simulink model "KukaSimModel"  (R2024b)
settings: Solver=VariableStepAuto  StartTime=0.0  StopTime=30  FixedStep=0.01  RelTol=1e-3
PreLoadFcn:
  | TP_TASK_SPACE = Simulink.Variant('TP_MODE==1');
  | TP_JOINT_SPACE = Simulink.Variant('TP_MODE==2');
InitFcn:
  | printlog('Start simulation...');
  | 
  | if TP_MODE == 1
  |     printlog('Run simulation...');
  |     return;
  | end
  | 
  | printlog('Solve Inverse Kinematics in JointSpace...');
  | jointWaypoints = zeros(6, size(waypointsStruct.waypoints, 2));
  | for i=1:size(waypointsStruct.waypoints, 2)
  |     if isempty(waypointsStruct.orientations)
  |         R = eye(3, 3);
  |     else
  |         R = trajectory.convertEulerToRotationMatrix(waypointsStruct.orientations(:, i));
  |     end
  |     % create homogeneous transform for inverse kinematics
  |     T = [R, waypointsStruct.waypoints(:, i); zeros(1, 3), 1];
  |     jointWaypoints(:, i) = solver.solveInverseKinematics(dhParametersStruct, T);
  | end
  | printlog('Run simulation...');
StopFcn:
  | t = datetime('now');
  | printlog('Stop simulation.');
undefined symbols (not defined in the file): dhParametersStruct, dt_FixedStep, dynamicParametersStruct, q1, q2, q3, q4, q5, q6, tau1, tau2, tau3, tau4, tau5, tau6, waypointsStruct
libraries: lib_Solver x5
settings Model: Creator=chiar  LastModifiedBy=Collins
settings OptimizationCC: BlockReduction=off  DefaultParameterBehavior=Inlined  BufferReuse=off
settings DebuggingCC: UnconnectedInputMsg=warning  UnconnectedOutputMsg=warning  UnconnectedLineMsg=warning
settings ModelReferenceCC: EnableRefExpFcnMdlSchedulingChecks=on
settings RTWCC: GPUComputeCapability=3.5  DLArmComputeVersion=19.05
settings GRTTargetCC: RTWCAPISignals=on  RTWCAPIParams=on

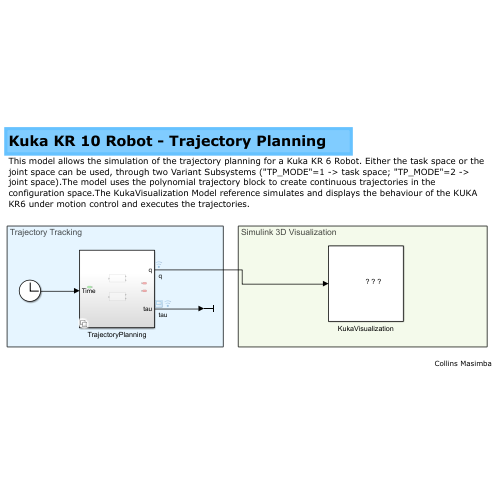
[thumbnail: Simulink's stored preview of the top-level diagram]
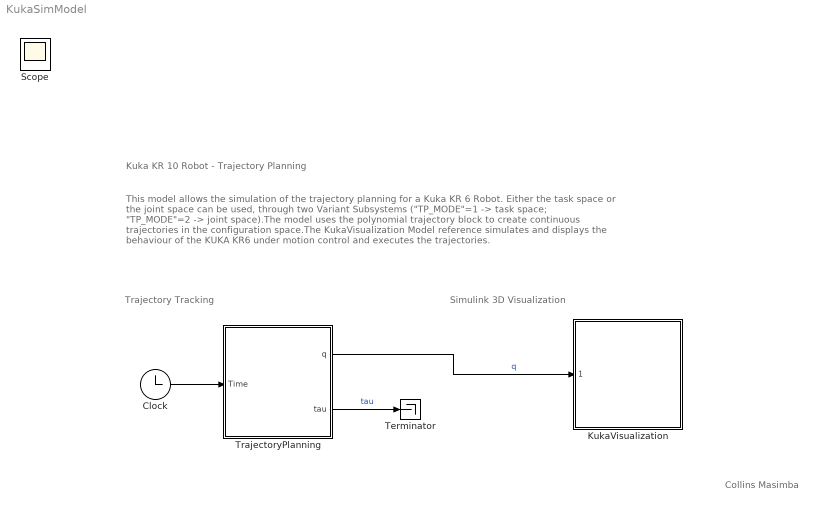
== system KukaSimModel ==
  note: Collins Masimba
  note: Trajectory Tracking
  note: Simulink 3D Visualization
  note: This model allows the simulation of the trajectory planning for a Kuka KR 6 Robot. Either the task space or the joint space can be used, through two Variant Subsystems ("TP_MODE"=1 -> task space; "TP_MODE"=2 -> joint space).The model uses the polynomial trajectory block to create continuous trajectories in the configuration space.The KukaVisualization Model reference simulates and displays the behaviour of the KUKA KR6 under motion control and executes the trajectories.
  note: Kuka KR 10 Robot - Trajectory Planning
  Clock : Clock
  KukaVisualization : Subsystem  ReferencedSubsystem=KukaVisualizationModel
  Terminator : Terminator
  TrajectoryPlanning : Subsystem  Variant=on
  Scope : Scope
  wires:
  TrajectoryPlanning/1(q) -> KukaVisualization/1  "q"
  Clock/1 -> TrajectoryPlanning/1(Time)
  TrajectoryPlanning/2(tau) -> Terminator/1  "tau"

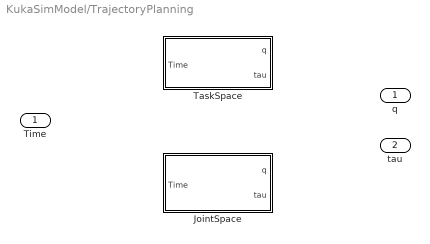
== system KukaSimModel/TrajectoryPlanning ==
  Time : Inport
  JointSpace : Subsystem  VariantControl=TP_MODE == 2
  TaskSpace : Subsystem  VariantControl=TP_MODE == 1
  q : Outport  OutDataTypeStr=Bus: Bus_q
  tau : Outport  Port=2  OutDataTypeStr=double

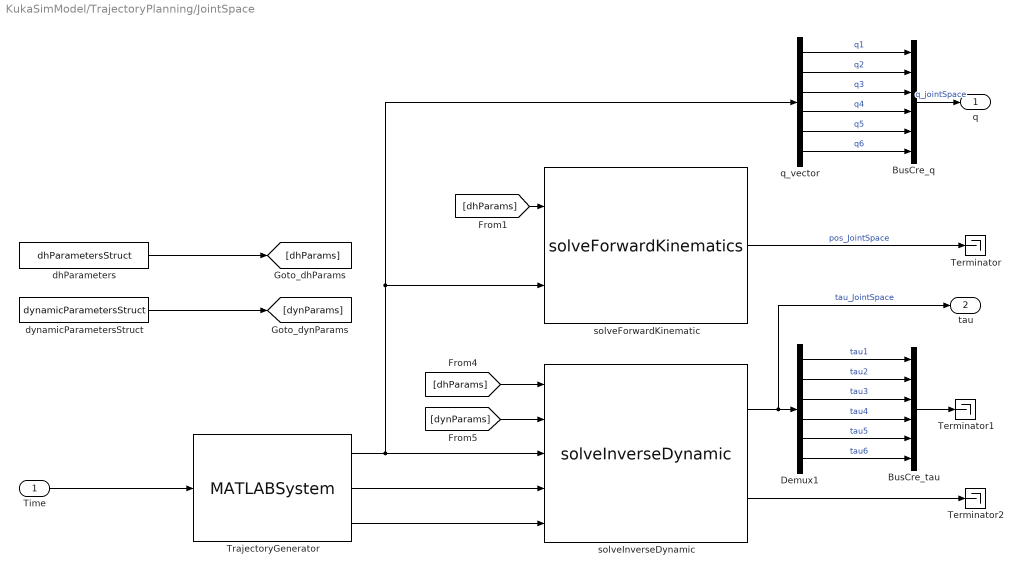
== system KukaSimModel/TrajectoryPlanning/JointSpace ==
  Time : Inport
  BusCre_q : BusCreator  Inputs=q1,q2,q3,q4,q5,q6  OutDataTypeStr=Bus: Bus_q
  BusCre_tau : BusCreator  Inputs=tau1,tau2,tau3,tau4,tau5,tau6  OutDataTypeStr=Bus: Bus_tau
  Demux1 : Demux  Outputs=6
  Terminator : Terminator
  Terminator1 : Terminator
  Terminator2 : Terminator
  TrajectoryGenerator : MATLABSystem  System=core.TrajectoryGenerator  SolverSpace=JointSpace  Method=Cubic Polynomial  Waypoints=jointWaypoints  Timepoints=waypointsStruct.times  Velocities=zeros(6, size(waypointsStruct.waypoints, 2))  Accelerations=zeros(6, size(waypointsStruct.waypoints, 2))  Orientations=zeros( 3, 5 )  PropertyLogical=off  SimulateUsing=Interpreted execution
  dhParameters : Constant  Value=dhParametersStruct  OutDataTypeStr=Bus: Bus_dhParameter
  dynamicParametersStruct : Constant  Value=dynamicParametersStruct  OutDataTypeStr=Bus: Bus_dynamicsParameter
  q_vector : Demux  Outputs=6
  solveForwardKinematic : lib_Solver/solveForwardKinematics  SystemSampleTime=-1  VariantActivationTime=update diagram  Latency=0  AutoFrameSizeCalculation=off
  solveInverseDynamic : lib_Solver/solveInverseDynamic  SystemSampleTime=-1  VariantActivationTime=update diagram  Latency=0  AutoFrameSizeCalculation=off
  q : Outport  OutDataTypeStr=Bus: Bus_q
  tau : Outport  Port=2  OutDataTypeStr=double
  wires:
  Time/1 -> TrajectoryGenerator/1
  [dynParams] -> solveInverseDynamic/2
  [dhParams] -> solveInverseDynamic/1
  solveInverseDynamic/1 -> tau/1, Demux1/1  "tau_JointSpace"
  q_vector/6 -> BusCre_q/6  "q6"
  q_vector/1 -> BusCre_q/1  "q1"
  q_vector/2 -> BusCre_q/2  "q2"
  q_vector/3 -> BusCre_q/3  "q3"
  q_vector/5 -> BusCre_q/5  "q5"
  q_vector/4 -> BusCre_q/4  "q4"
  TrajectoryGenerator/1 -> solveInverseDynamic/3, q_vector/1, solveForwardKinematic/2
  BusCre_q/1 -> q/1  "q_jointSpace"
  solveInverseDynamic/2 -> Terminator2/1
  dhParameters/1 -> [dhParams]
  dynamicParametersStruct/1 -> [dynParams]
  [dhParams] -> solveForwardKinematic/1
  solveForwardKinematic/1 -> Terminator/1  "pos_JointSpace"
  TrajectoryGenerator/2 -> solveInverseDynamic/4
  TrajectoryGenerator/3 -> solveInverseDynamic/5
  Demux1/4 -> BusCre_tau/4  "tau4"
  Demux1/5 -> BusCre_tau/5  "tau5"
  Demux1/3 -> BusCre_tau/3  "tau3"
  Demux1/1 -> BusCre_tau/1  "tau1"
  Demux1/6 -> BusCre_tau/6  "tau6"
  Demux1/2 -> BusCre_tau/2  "tau2"
  BusCre_tau/1 -> Terminator1/1

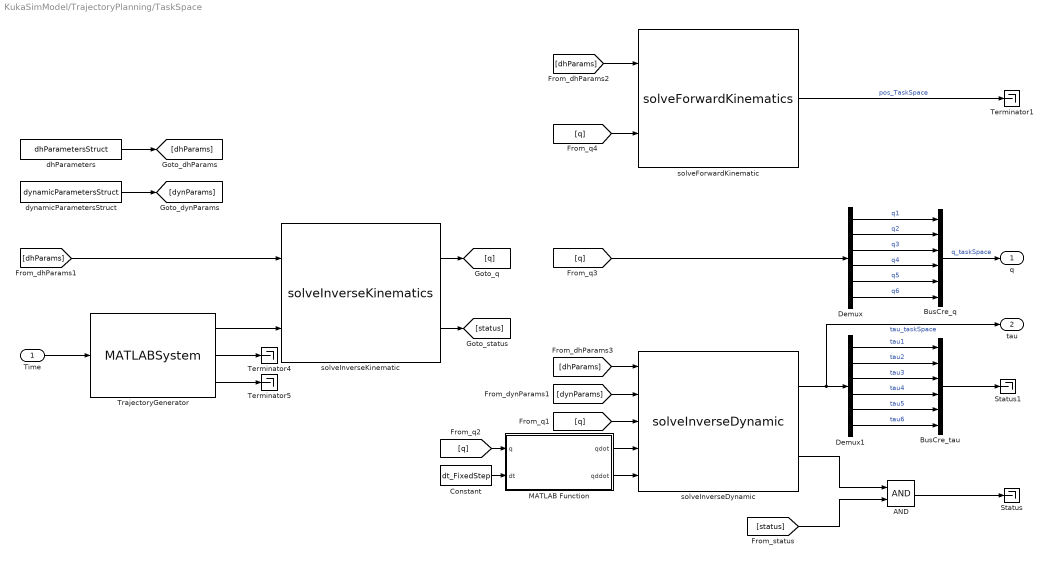
== system KukaSimModel/TrajectoryPlanning/TaskSpace ==
  Time : Inport
  AND : Logic  AllPortsSameDT=off  OutDataTypeStr=boolean
  BusCre_q : BusCreator  Inputs=q1,q2,q3,q4,q5,q6  OutDataTypeStr=Bus: Bus_q
  BusCre_tau : BusCreator  Inputs=tau1,tau2,tau3,tau4,tau5,tau6  OutDataTypeStr=Bus: Bus_tau
  Constant : Constant  Value=dt_FixedStep  OutDataTypeStr=double
  Demux : Demux  Outputs=6
  Demux1 : Demux  Outputs=6
  MATLAB Function : MATLAB Function  TreatAsAtomicUnit=on
  Status : Terminator
  Status1 : Terminator
  Terminator1 : Terminator
  Terminator4 : Terminator
  Terminator5 : Terminator
  TrajectoryGenerator : MATLABSystem  System=core.TrajectoryGenerator  SolverSpace=JointSpace  Method=Quintic Polynomial  Waypoints=waypointsStruct.waypoints  Timepoints=waypointsStruct.times  Velocities=waypointsStruct.velocities  Accelerations=waypointsStruct.accelerations  Orientations=waypointsStruct.orientations  PropertyLogical=off  SimulateUsing=Interpreted execution
  dhParameters : Constant  Value=dhParametersStruct  OutDataTypeStr=Bus: Bus_dhParameter
  dynamicParametersStruct : Constant  Value=dynamicParametersStruct  OutDataTypeStr=Bus: Bus_dynamicsParameter
  solveForwardKinematic : lib_Solver/solveForwardKinematics  SystemSampleTime=-1  VariantActivationTime=update diagram  Latency=0  AutoFrameSizeCalculation=off
  solveInverseDynamic : lib_Solver/solveInverseDynamic  SystemSampleTime=-1  VariantActivationTime=update diagram  Latency=0  AutoFrameSizeCalculation=off
  solveInverseKinematic : lib_Solver/solveInverseKinematics  SystemSampleTime=-1  VariantActivationTime=update diagram  Latency=0  AutoFrameSizeCalculation=off
  q : Outport  OutDataTypeStr=Bus: Bus_q
  tau : Outport  Port=2  OutDataTypeStr=double
  wires:
  Time/1 -> TrajectoryGenerator/1
  solveInverseDynamic/1 -> tau/1, Demux1/1  "tau_taskSpace"
  TrajectoryGenerator/2 -> Terminator4/1
  TrajectoryGenerator/3 -> Terminator5/1
  Demux/1 -> BusCre_q/1  "q1"
  Demux/2 -> BusCre_q/2  "q2"
  Demux/3 -> BusCre_q/3  "q3"
  Demux/4 -> BusCre_q/4  "q4"
  Demux/5 -> BusCre_q/5  "q5"
  Demux/6 -> BusCre_q/6  "q6"
  BusCre_q/1 -> q/1  "q_taskSpace"
  solveInverseDynamic/2 -> AND/1
  AND/1 -> Status/1
  [status] -> AND/2
  solveInverseKinematic/2 -> [status]
  dhParameters/1 -> [dhParams]
  [dhParams] -> solveForwardKinematic/1
  [dhParams] -> solveInverseDynamic/1
  [dynParams] -> solveInverseDynamic/2
  dynamicParametersStruct/1 -> [dynParams]
  [dhParams] -> solveInverseKinematic/1
  TrajectoryGenerator/1 -> solveInverseKinematic/2
  MATLAB Function/2(qddot) -> solveInverseDynamic/5
  MATLAB Function/1(qdot) -> solveInverseDynamic/4
  Constant/1 -> MATLAB Function/2(dt)
  solveForwardKinematic/1 -> Terminator1/1  "pos_TaskSpace"
  solveInverseKinematic/1 -> [q]
  [q] -> MATLAB Function/1(q)
  [q] -> solveInverseDynamic/3
  [q] -> Demux/1
  [q] -> solveForwardKinematic/2
  Demux1/6 -> BusCre_tau/6  "tau6"
  Demux1/3 -> BusCre_tau/3  "tau3"
  Demux1/5 -> BusCre_tau/5  "tau5"
  Demux1/2 -> BusCre_tau/2  "tau2"
  Demux1/4 -> BusCre_tau/4  "tau4"
  Demux1/1 -> BusCre_tau/1  "tau1"
  BusCre_tau/1 -> Status1/1

== matlab function KukaSimModel/TrajectoryPlanning/TaskSpace/MATLAB Function ==
  data: q input; qdot output; dt input; qddot output
function [qdot, qddot] = calculateGradient(q, dt)

qdot = gradient(q, dt);
qddot = gradient(qdot, dt);
